simulink model "PosFBGenerator"  (Simulink 10.2)
settings: Solver=ode45  StartTime=0.0  StopTime=5  RelTol=1e-3  EnableMultiTasking=on
libraries: NeuroModelerLibrary x4
settings Model: Creator=Bakhshiev  LastModifiedBy=Bakhshiev
settings DataIOCC: LimitDataPoints=on
settings OptimizationCC: ExpressionDepthLimit=2147483647
settings DebuggingCC: SolverPrmCheckMsg=warning  StateNameClashWarn=warning
settings ConfigComp: CovSFcnEnable=off

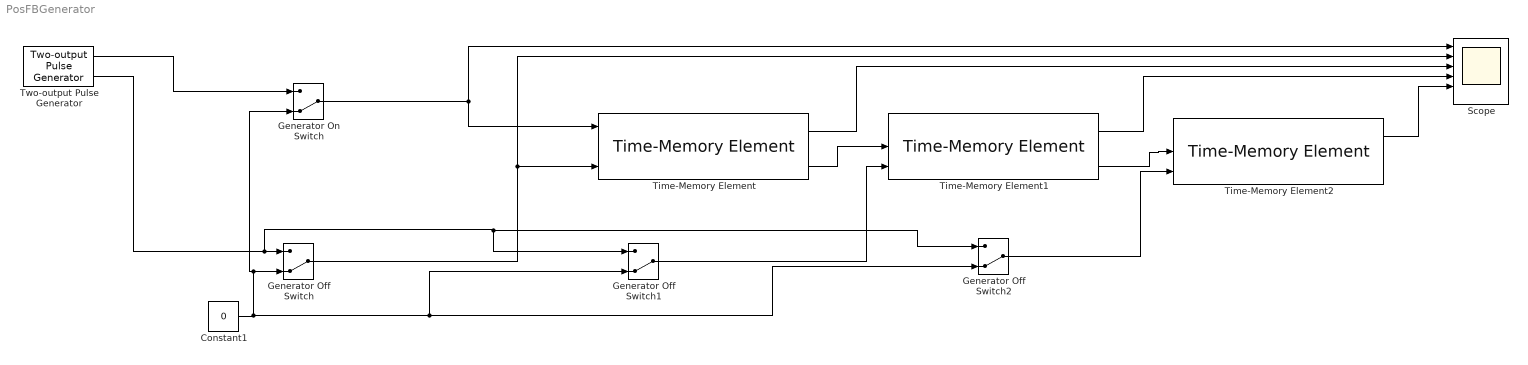
== system PosFBGenerator ==
  Constant1 : Constant  Value=0
  Generator Off Switch : ManualSwitch  CurrentSetting=0
  Generator Off Switch1 : ManualSwitch  CurrentSetting=0
  Generator Off Switch2 : ManualSwitch  CurrentSetting=0
  Generator On Switch : ManualSwitch  CurrentSetting=0
  Scope : Scope  NumInputPorts=6
  Time-Memory Element : NeuroModelerLibrary/Memory Modules/Time-Memory Element  SystemSampleTime=-1  VariantActivationTime=update diagram  Latency=0  AutoFrameSizeCalculation=off
  Time-Memory Element1 : NeuroModelerLibrary/Memory Modules/Time-Memory Element  SystemSampleTime=-1  VariantActivationTime=update diagram  Latency=0  AutoFrameSizeCalculation=off
  Time-Memory Element2 : NeuroModelerLibrary/Memory Modules/Time-Memory Element  SystemSampleTime=-1  VariantActivationTime=update diagram  Latency=0  AutoFrameSizeCalculation=off
  Two-output Pulse Generator : NeuroModelerLibrary/Support/Two-output Pulse Generator  A=1  P1=1000  P2=30  PW=1  ST=0.001  OOn1=0  OOff1=7700  OOn2=0  OOff2=7000
  wires:
  Two-output Pulse Generator/1 -> Generator On Switch/1
  Constant1/1 -> Generator Off Switch2/2, Generator Off Switch1/2, Generator On Switch/2, Generator Off Switch/2
  Two-output Pulse Generator/2 -> Generator Off Switch2/1, Generator Off Switch1/1, Generator Off Switch/1
  Generator On Switch/1 -> Time-Memory Element/1, Scope/1
  Generator Off Switch/1 -> Time-Memory Element/3, Scope/2
  Time-Memory Element/1 -> Scope/3
  Time-Memory Element/2 -> Time-Memory Element1/2
  Time-Memory Element1/2 -> Time-Memory Element2/2
  Time-Memory Element1/1 -> Scope/4
  Time-Memory Element2/1 -> Scope/5
  Generator Off Switch1/1 -> Time-Memory Element1/3
  Generator Off Switch2/1 -> Time-Memory Element2/3
